simulink model "EV_Controller"  (R2026a)
settings: Solver=VariableStepAuto
settings Model: Creator=chowdeswara.rao  LastModifiedBy=chowdeswara.rao

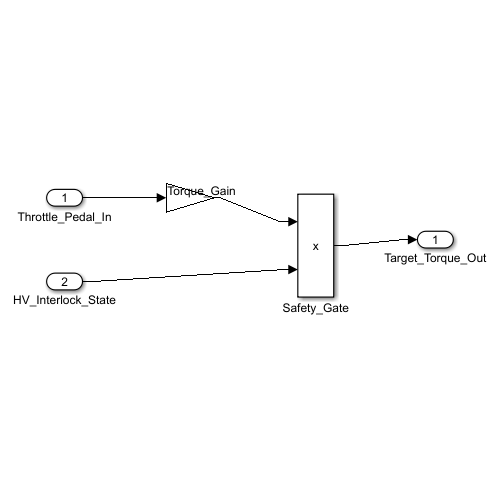
[thumbnail: Simulink's stored preview of the top-level diagram]
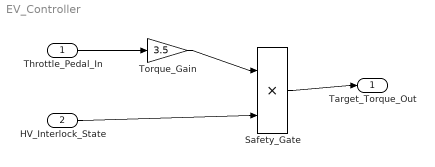
== system EV_Controller ==
  Throttle_Pedal_In : Inport
  HV_Interlock_State : Inport  Port=2
  Safety_Gate : Product
  Torque_Gain : Gain  Gain=3.5
  Target_Torque_Out : Outport
  wires:
  Throttle_Pedal_In/1 -> Torque_Gain/1
  Torque_Gain/1 -> Safety_Gate/1
  HV_Interlock_State/1 -> Safety_Gate/2
  Safety_Gate/1 -> Target_Torque_Out/1
